simulink model "task2"  (R2018a)
settings: Solver=ode45  StartTime=0.0  StopTime=5000  RelTol=1e-3  EnableMultiTasking=on
settings Model: Creator=Альбнка-Ноут  LastModifiedBy=User
settings DataIOCC: LimitDataPoints=on  SaveFormat=Array  SignalLoggingSaveFormat=ModelDataLogs
settings OptimizationCC: LifeSpan=inf
settings DebuggingCC: MultiTaskDSMMsg=warning  MultiTaskCondExecSysMsg=none  SFUnexpectedBacktrackingDiag=warning  SFNoUnconditionalDefaultTransitionDiag=warning  SFExecutionAtInitializationDiag=none
settings HardwareCC: ProdBitPerPointer=32  ProdBitPerSizeT=32  ProdBitPerPtrDiffT=32  ProdLargestAtomicFloat=None  ProdIntDivRoundTo=Undefined  ProdEndianess=Unspecified  ProdWordSize=32  ProdHWDeviceType=32-bit Generic
settings ModelReferenceCC: PropagateSignalLabelsOutOfModel=off
settings CodeAppCC: StateflowObjectComments=on
settings GRTTargetCC: TargetLangStandard=C89/C90 (ANSI)  GeneratePreprocessorConditionals=Disable all
settings ConfigComp: CovMetricSettings=dw  CovHtmlReporting=on  CovSaveCumulativeToWorkspaceVar=on  CovSaveSingleToWorkspaceVar=on  CovExternalEMLEnable=off  CovSFcnEnable=off

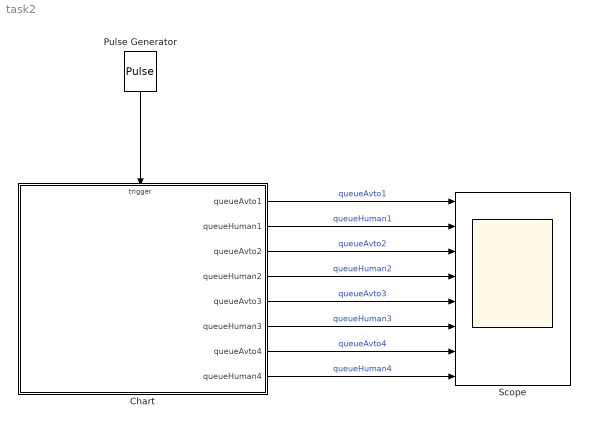
== system task2 ==
  Chart : Stateflow chart  TreatAsAtomicUnit=on
  Pulse Generator : DiscretePulseGenerator  PulseType=Time based  Period=1  PulseWidth=5
  Scope : Scope  NumInputPorts=8
  wires:
  Pulse Generator/1 -> Chart/Trigger
  Chart/1(queueAvto1) -> Scope/1  "queueAvto1"
  Chart/2(queueHuman1) -> Scope/2  "queueHuman1"
  Chart/3(queueAvto2) -> Scope/3  "queueAvto2"
  Chart/4(queueHuman2) -> Scope/4  "queueHuman2"
  Chart/5(queueAvto3) -> Scope/5  "queueAvto3"
  Chart/6(queueHuman3) -> Scope/6  "queueHuman3"
  Chart/7(queueAvto4) -> Scope/7  "queueAvto4"
  Chart/8(queueHuman4) -> Scope/8  "queueHuman4"

== stateflow chart task2/Chart ==
  state GeneratorAvto2/ [parallel]
    settings: executionOrder=6
    state vihod/
      entry:queueAvto2++;
    state generatorAvto2/
    (default) -> generatorAvto2 : /timeAvto2=0;
        | queueAvto2=0;
    generatorAvto2 -> GeneratorAvto2.vihod : after(60,sec)
    GeneratorAvto2.vihod -> generatorAvto2
  state GeneratorHuman2/ [parallel]
    settings: executionOrder=7
    state vihod/
      entry:queueHuman2++;
    state generatorHuman2/
    (default) -> generatorHuman2 : /timeHuman2=0;
        | queueHuman2=0;
    generatorHuman2 -> GeneratorHuman2.vihod : after(30,sec)
    GeneratorHuman2.vihod -> generatorHuman2
  state serverAvto2/ [parallel]
    settings: executionOrder=8
    state vhod/
    state directionAvto2/
      entry:directionAvto2=ml('randi(101)-1');
    state avto2Straight/
      entry:
      timeServerAvto2=ml('unifrnd(5,10)')
      workServerAvto2Straight=1
      exit:
      workServerAvto2Straight=0
    state ServerAvto2Left/
      entry:
      timeServerAvto2=ml('unifrnd(5,10)')
      workServerAvto2Left=1
      exit:
      workServerAvto2Left=0
    state avto2Right/
      entry:
      timeServerAvto2=ml('unifrnd(5,10)')
      workServerAvto2Right=1
      exit:
      workServerAvto2Right=0
    (default) -> serverAvto2.vhod : /timeServerAvto2=0
    (junction 2231) -> serverAvto2.vhod : {queueAvto2--;}
    (junction 2208) -> (junction 2231)
    serverAvto2.vhod -> directionAvto2 : [queueAvto2>0 && ...
        | Light2==1]
    directionAvto2 -> ServerAvto2Left [order 1] : [directionAvto2<(33) && ...
        | workServerAvto1Straight==0 && ...
        | workServerAvto1Right==0 && ...
        | workServerHuman1==0]
    directionAvto2 -> avto2Straight [order 2] : [directionAvto2>=(33) && directionAvto2<(67)]
    directionAvto2 -> avto2Right [order 3] : [directionAvto2>=(67) && ...
        | workServerHuman2==0]
    avto2Right -> (junction 2205) : after(timeServerAvto2,sec)
    ServerAvto2Left -> (junction 2204) : after(timeServerAvto2,sec)
    avto2Straight -> (junction 2226) : after(timeServerAvto2,sec)
    (junction 2204) -> (junction 2226)
    (junction 2226) -> (junction 2205)
    (junction 2205) -> (junction 2208)
  state serverHuman2/ [parallel]
    settings: executionOrder=9
    state vhod/
    state Human2/
      entry:
      timeServerHuman2=ml('unifrnd(5,10)')
      workServerHuman2=1
      exit:
      workServerHuman2=0
    (default) -> serverHuman2.vhod
    (junction 2222) -> serverHuman2.vhod : {queueHuman2--;}
    (junction 2213) -> (junction 2222)
    serverHuman2.vhod -> Human2 : [workServerAvto2Right==0 && ...
        | workServerAvto1Left==0 && ...
        | queueHuman2>0 && ...
        | Light2==1]
    Human2 -> (junction 2215) : after(timeServerAvto2,sec)
    (junction 2215) -> (junction 2213)
  state GeneratorAvto4/ [parallel]
    settings: executionOrder=16
    state vihod/
      entry:queueAvto4++;
    state generatorAvto4/
    (default) -> generatorAvto4 : /timeAvto4=0;
        | queueAvto4=0;
    generatorAvto4 -> GeneratorAvto4.vihod : after(60,sec)
    GeneratorAvto4.vihod -> generatorAvto4
  state serverAvto4/ [parallel]
    settings: executionOrder=18
    state vhod/
    state directionAvto4/
      entry:directionAvto4=ml('randi(101)-1');
    state avto4Straight/
      entry:
      timeServerAvto4=ml('unifrnd(5,10)')
      workServerAvto4Straight=1
      exit:
      workServerAvto4Straight=0
    state ServerAvto4Left/
      entry:
      timeServerAvto4=ml('unifrnd(5,10)')
      workServerAvto4Left=1
      exit:
      workServerAvto4Left=0
    state avto4Right/
      entry:
      timeServerAvto4=ml('unifrnd(5,10)')
      workServerAvto4Right=1
      exit:
      workServerAvto4Right=0
    (default) -> serverAvto4.vhod : /timeServerAvto4=0
    (junction 2460) -> serverAvto4.vhod : {queueAvto4--;}
    (junction 2424) -> (junction 2460)
    serverAvto4.vhod -> directionAvto4 : [queueAvto4>0 && ...
        | Light4==1]
    directionAvto4 -> ServerAvto4Left [order 1] : [directionAvto4<(33) && ...
        | workServerAvto3Straight==0 && ...
        | workServerAvto3Right==0 && ...
        | workServerHuman3==0]
    directionAvto4 -> avto4Straight [order 2] : [directionAvto43>=(33) && directionAvto4<(67)]
    directionAvto4 -> avto4Right [order 3] : [directionAvto1>=(67) && ...
        | workServerHuman1==0]
    avto4Right -> (junction 2433) : after(timeServerAvto4,sec)
    ServerAvto4Left -> (junction 2431) : after(timeServerAvto4,sec)
    avto4Straight -> (junction 2436) : after(timeServerAvto4,sec)
    (junction 2431) -> (junction 2436)
    (junction 2436) -> (junction 2433)
    (junction 2433) -> (junction 2424)
  state GeneratorAvto3/ [parallel]
    settings: executionOrder=11
    state vihod/
      entry:queueAvto3++;
    state generatorAvto3/
    (default) -> generatorAvto3 : /timeAvto3=0;
        | queueAvto3=0;
    generatorAvto3 -> GeneratorAvto3.vihod : after(60,sec)
    GeneratorAvto3.vihod -> generatorAvto3
  state serverAvto3/ [parallel]
    settings: executionOrder=13
    state vhod/
    state directionAvto3/
      entry:directionAvto3=ml('randi(101)-1');
    state avto3Straight/
      entry:
      timeServerAvto3=ml('unifrnd(5,10)')
      workServerAvto3Straight=1
      exit:
      workServerAvto3Straight=0
    state ServerAvto3Left/
      entry:
      timeServerAvto3=ml('unifrnd(5,10)')
      workServerAvto3Left=1
      exit:
      workServerAvto3Left=0
    state avto3Right/
      entry:
      timeServerAvto3=ml('unifrnd(5,10)')
      workServerAvto3Right=1
      exit:
      workServerAvto3Right=0
    (default) -> serverAvto3.vhod : /timeServerAvto3=0
    (junction 2333) -> serverAvto3.vhod : {queueAvto3--;}
    (junction 2310) -> (junction 2333)
    serverAvto3.vhod -> directionAvto3 : [queueAvto3>0 && ...
        | Light3==1]
    directionAvto3 -> ServerAvto3Left [order 1] : [directionAvto3<(33) && ...
        | workServerAvto4Straight==0 && ...
        | workServerAvto4Right==0 && ...
        | workServerHuman4==0]
    directionAvto3 -> avto3Straight [order 2] : [directionAvto3>=(33) && directionAvto3<(67)]
    directionAvto3 -> avto3Right [order 3] : [directionAvto1>=(67) && ...
        | workServerHuman1==0]
    avto3Right -> (junction 2307) : after(timeServerAvto3,sec)
    ServerAvto3Left -> (junction 2306) : after(timeServerAvto3,sec)
    avto3Straight -> (junction 2328) : after(timeServerAvto3,sec)
    (junction 2306) -> (junction 2328)
    (junction 2328) -> (junction 2307)
    (junction 2307) -> (junction 2310)
  state Svetofor2/ [parallel]
    settings: executionOrder=10
    state Green2/
      entry:
      Light2=1
    state Yellow2/
      entry:
      Light2=2
    state Red2/
      entry:
      Light2=3
    Red2 -> Green2 : after(40,sec)
    Yellow2 -> Red2 : after(10,sec)
    Green2 -> Yellow2 : after(30,sec)
    (default) -> Green2 : /Light2=1
  state Svetofor3/ [parallel]
    settings: executionOrder=15
    state Red3/
      entry:
      Light3=3
    state Yellow3/
      entry:
      Light3=2
    state Green3/
      entry:
      Light3=1
    (default) -> Red3 : /Light3=3
    Red3 -> Green3 : after(40,sec)
    Yellow3 -> Red3 : after(10,sec)
    Green3 -> Yellow3 : after(30,sec)
  state Svetofor4/ [parallel]
    settings: executionOrder=20
    state Red4/
      entry:
      Light4=3
    state Yellow4/
      entry:
      Light4=2
    state Green4/
      entry:
      Light4=1
    (default) -> Red4 : /Light4=3
    Red4 -> Green4 : after(40,sec)
    Yellow4 -> Red4 : after(10,sec)
    Green4 -> Yellow4 : after(30,sec)
  state serverHuman4/ [parallel]
    settings: executionOrder=19
    state vhod/
    state Human4/
      entry:
      timeServerHuman4=ml('unifrnd(5,10)')
      workServerHuman4=1
      exit:
      workServerHuman4=0
    (default) -> serverHuman4.vhod
    (junction 2459) -> serverHuman4.vhod : {queueHuman4--;}
    (junction 2430) -> (junction 2459)
    serverHuman4.vhod -> Human4 : [workServerAvto4Right==0 && ...
        | workServerAvto3Left==0 && ...
        | queueHuman4>0 && ...
        | Light4==1]
    Human4 -> (junction 2412) : after(timeServerAvto4,sec)
    (junction 2412) -> (junction 2430)
  state GeneratorHuman4/ [parallel]
    settings: executionOrder=17
    state vihod/
      entry:queueHuman4++;
    state generatorHuman4/
    (default) -> generatorHuman4 : /timeHuman4=0;
        | queueHuman4=0;
    generatorHuman4 -> GeneratorHuman4.vihod : after(30,sec)
    GeneratorHuman4.vihod -> generatorHuman4
  state serverHuman3/ [parallel]
    settings: executionOrder=14
    state vhod/
    state Human3/
      entry:
      timeServerHuman3=ml('unifrnd(5,10)')
      workServerHuman3=1
      exit:
      workServerHuman3=0
    (default) -> serverHuman3.vhod
    (junction 2324) -> serverHuman3.vhod : {queueHuman3--;}
    (junction 2315) -> (junction 2324)
    serverHuman3.vhod -> Human3 : [workServerAvto3Right==0 && ...
        | workServerAvto4Left==0 && ...
        | queueHuman3>0 && ...
        | Light3==1]
    Human3 -> (junction 2317) : after(timeServerAvto3,sec)
    (junction 2317) -> (junction 2315)
  state GeneratorHuman3/ [parallel]
    settings: executionOrder=12
    state vihod/
      entry:queueHuman3++;
    state generatorHuman3/
    (default) -> generatorHuman3 : /timeHuman3=0;
        | queueHuman3=0;
    generatorHuman3 -> GeneratorHuman3.vihod : after(30,sec)
    GeneratorHuman3.vihod -> generatorHuman3
  state Svetofor1/ [parallel]
    settings: executionOrder=5
    state Green1/
      entry:
      Light1=1
    state Yellow1/
      entry:
      Light1=2
    state Red1/
      entry:
      Light1=3
    Yellow1 -> Red1 : after(10,sec)
    Green1 -> Yellow1 : after(30,sec)
    (default) -> Green1 : /Light1=1
    Red1 -> Green1 : after(40,sec)
  state serverAvto1/ [parallel]
    settings: executionOrder=3
    state vhod/
    state directionAvto1/
      entry:directionAvto1=ml('randi(101)-1');
    state avto1Straight/
      entry:
      timeServerAvto1=ml('unifrnd(5,10)')
      workServerAvto1Straight=1
      exit:
      workServerAvto1Straight=0
    state ServerAvto1Left/
      entry:
      timeServerAvto1=ml('unifrnd(5,10)')
      workServerAvto1Left=1
      exit:
      workServerAvto1Left=0
    state avto1Right/
      entry:
      timeServerAvto1=ml('unifrnd(5,10)')
      workServerAvto1Right=1
      exit:
      workServerAvto1Right=0
    (default) -> serverAvto1.vhod : /timeServerAvto1=0
    (junction 2092) -> serverAvto1.vhod : {queueAvto1--;}
    (junction 2101) -> (junction 2092)
    serverAvto1.vhod -> directionAvto1 : [queueAvto1>0 && ...
        | Light1==1]
    directionAvto1 -> ServerAvto1Left [order 1] : [directionAvto1<(33) && ...
        | workServerAvto2Straight==0 && ...
        | workServerAvto2Right==0 && ...
        | workServerHuman2==0]
    directionAvto1 -> avto1Straight [order 2] : [directionAvto1>=(33) && directionAvto1<(67)]
    directionAvto1 -> avto1Right [order 3] : [directionAvto1>=(67) && ...
        | workServerHuman1==0]
    avto1Right -> (junction 2098) : after(timeServerAvto1,sec)
    ServerAvto1Left -> (junction 2095) : after(timeServerAvto1,sec)
    avto1Straight -> (junction 2086) : after(timeServerAvto1,sec)
    (junction 2095) -> (junction 2086)
    (junction 2086) -> (junction 2098)
    (junction 2098) -> (junction 2101)
  state serverHuman1/ [parallel]
    settings: executionOrder=4
    state vhod/
    state Human1/
      entry:
      timeServerHuman1=ml('unifrnd(5,10)')
      workServerHuman1=1
      exit:
      workServerHuman1=0
    (default) -> serverHuman1.vhod
    (junction 2123) -> serverHuman1.vhod : {queueHuman1--;}
    (junction 2111) -> (junction 2123)
    serverHuman1.vhod -> Human1 : [workServerAvto1Right==0 && ...
        | workServerAvto2Left==0 && ...
        | queueHuman1>0 && ...
        | Light1==1]
    Human1 -> (junction 2118) : after(timeServerAvto1,sec)
    (junction 2118) -> (junction 2111)
  state GeneratorHuman1/ [parallel]
    settings: executionOrder=2
    state vihod/
      entry:queueHuman1++;
    state generatorHuman1/
    (default) -> generatorHuman1 : /timeHuman1=0;
        | queueHuman1=0;
    generatorHuman1 -> GeneratorHuman1.vihod : after(30,sec)
    GeneratorHuman1.vihod -> generatorHuman1
  state GeneratorAvto1/ [parallel]
    settings: executionOrder=1
    state vihod/
      entry:queueAvto1++;
    state generatorAvto1/
    (default) -> generatorAvto1 : /timeAvto1=0;
        | queueAvto1=0;
    generatorAvto1 -> GeneratorAvto1.vihod : after(60,sec)
    GeneratorAvto1.vihod -> generatorAvto1
  data: timeAvto1 local double; timeHuman1 local double; directionAvto1 local double; timeServerAvto1 local double; workServerAvto1Left local double; workServerAvto1Right local double; workServerAvto1Straight local double; workServerHuman local double; timeServerHuman1 local double; workServerHuman1 local double; Light1 local double; Light2 local double; timeAvto2 local double; timeHuman2 local double; timeServerHuman2 local double; directionAvto2 local double; timeServerAvto2 local double; workServerAvto2Left local double; workServerAvto2Right local double; workServerAvto2Straight local double; workServerHuman2 local double; Light3 local double; queueAvto1 output double; queueHuman1 output double; queueAvto2 output double; queueHuman2 output double; directionAvto43 local double; timeAvto3 local double; timeAvto4 local double; timeHuman3 local double; timeHuman4 local double; timeServerHuman3 local double; timeServerHuman4 local double; Light4 local double; directionAvto3 local double; directionAvto4 local double; timeServerAvto3 local double; timeServerAvto4 local double; workServerAvto3Left local double; workServerAvto3Right local double; workServerAvto3Straight local double; workServerAvto4Left local double; workServerAvto4Right local double; workServerAvto4Straight local double; workServerHuman3 local double; workServerHuman4 local double; queueAvto3 output double; queueHuman3 output double; queueAvto4 output double; queueHuman4 output double
  events: event input RISING_EDGE_EVENT
